simulink library "se2a_command_lib"  (R2018b)
settings: Solver=VariableStepAuto  StartTime=0.0  StopTime=10.0  RelTol=1e-3
undefined symbols (not defined in the file): aircraft
libraries: unit_conversions_lib x5, $bdroot x1
settings Model: Creator=Ybeyer  LastModifiedBy=cava_da
settings SFSimCC: SimUseLocalCustomCode=off
settings RTWCC: RTWUseLocalCustomCode=off
settings CodeAppCC: StateflowObjectComments=on

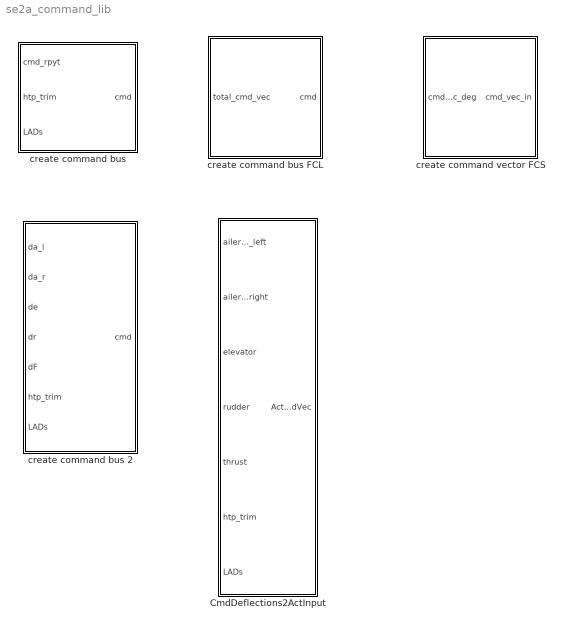
== system se2a_command_lib ==
  CmdDeflections2ActInput : Subsystem  mask{actuators=aircraft.actuators}
      mask prompts: actuators "Actuator parameters"
  create command bus : Subsystem  mask{num_ailerons=aircraft.wing_main.params.num_flaps/2}
      mask prompts: num_ailerons "Number of ailerons per side"
      mask DialogControl DescGroupVar Prompt: Create command bus
  create command bus 2 : Subsystem
      mask DialogControl DescGroupVar Prompt: Create command bus
  create command bus FCL : Subsystem  mask{n_ail_pairs=aircraft.wing_main.params.num_flaps/2, n_LADs=aircraft.wing_main.params.num_lads}
      mask prompts: n_ail_pairs "Number of aileron pairs"; n_LADs "Number of LADs"
      mask DialogControl DescGroupVar Prompt: Create command bus
  create command vector FCS : Subsystem  mask{n_ail_pairs=aircraft.wing_main.params.num_flaps/2, n_LADs=aircraft.wing_main.params.num_lads}
      mask prompts: n_ail_pairs "Number of aileron pairs"; n_LADs "Number of LADs"
      mask DialogControl DescGroupVar Prompt: Create command bus

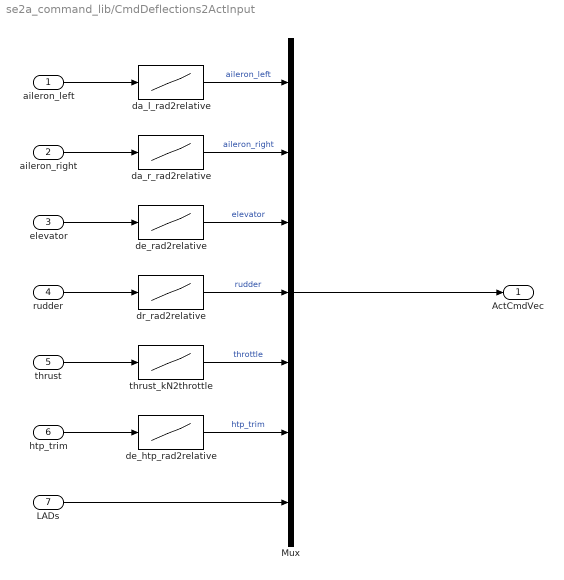
== system se2a_command_lib/CmdDeflections2ActInput ==
  aileron_left : Inport
  aileron_right : Inport  Port=2
  elevator : Inport  Port=3
  rudder : Inport  Port=4
  thrust : Inport  Port=5
  htp_trim : Inport  Port=6
  LADs : Inport  Port=7
  Mux : Mux  Inputs=7
  da_l_rad2relative : Lookup_n-D  NumberOfTableDimensions=1  BreakpointsForDimension1=[actuators.aileron.defl_min,actuators.aileron.defl_max]  Table=[-1,1]  ExtrapMethod=Clip  InternalRulePriority=Speed  RndMeth=Simplest  InputSameDT=on
  da_r_rad2relative : Lookup_n-D  NumberOfTableDimensions=1  BreakpointsForDimension1=[actuators.aileron.defl_min,actuators.aileron.defl_max]  Table=[-1,1]  ExtrapMethod=Clip  InternalRulePriority=Speed  RndMeth=Simplest  InputSameDT=on
  de_htp_rad2relative : Lookup_n-D  NumberOfTableDimensions=1  BreakpointsForDimension1=[actuators.htp_trim.defl_min,actuators.htp_trim.defl_max]  Table=[-1,1]  ExtrapMethod=Clip  InternalRulePriority=Speed  RndMeth=Simplest  InputSameDT=on
  de_rad2relative : Lookup_n-D  NumberOfTableDimensions=1  BreakpointsForDimension1=[actuators.elevator.defl_min,actuators.elevator.defl_max]  Table=[-1,1]  ExtrapMethod=Clip  InternalRulePriority=Speed  RndMeth=Simplest  InputSameDT=on
  dr_rad2relative : Lookup_n-D  NumberOfTableDimensions=1  BreakpointsForDimension1=[actuators.rudder.defl_min,actuators.rudder.defl_max]  Table=[-1,1]  ExtrapMethod=Clip  InternalRulePriority=Speed  RndMeth=Simplest  InputSameDT=on
  thrust_kN2throttle : Lookup_n-D  NumberOfTableDimensions=1  BreakpointsForDimension1=[0,actuators.engines.thrust_max]  Table=[0,1]  ExtrapMethod=Clip  InternalRulePriority=Speed  RndMeth=Simplest  InputSameDT=on
  ActCmdVec : Outport
  wires:
  LADs/1 -> Mux/7
  rudder/1 -> dr_rad2relative/1
  htp_trim/1 -> de_htp_rad2relative/1
  aileron_right/1 -> da_r_rad2relative/1
  Mux/1 -> ActCmdVec/1
  thrust/1 -> thrust_kN2throttle/1
  elevator/1 -> de_rad2relative/1
  de_rad2relative/1 -> Mux/3  "elevator"
  de_htp_rad2relative/1 -> Mux/6  "htp_trim"
  dr_rad2relative/1 -> Mux/4  "rudder"
  da_l_rad2relative/1 -> Mux/1  "aileron_left"
  thrust_kN2throttle/1 -> Mux/5  "throttle"
  da_r_rad2relative/1 -> Mux/2  "aileron_right"
  aileron_left/1 -> da_l_rad2relative/1

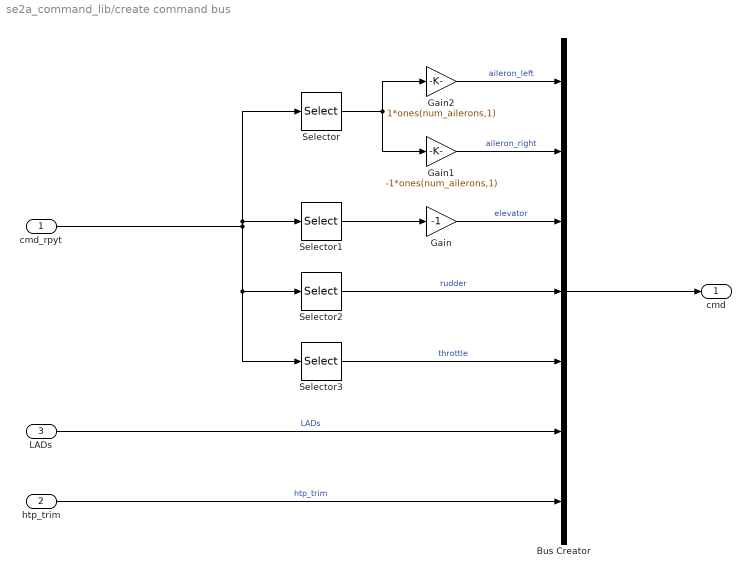
== system se2a_command_lib/create command bus ==
  cmd_rpyt : Inport
  htp_trim : Inport  Port=2
  LADs : Inport  Port=3
  Bus Creator : BusCreator  Inputs=7
  Gain : Gain  Gain=-1
  Gain1 : Gain  Gain=-1*ones(num_ailerons,1)
  Gain2 : Gain  Gain=1*ones(num_ailerons,1)
  Selector : Selector  InputPortWidth=4  IndexOptions=Index vector (dialog)  Indices=1  OutputSizes=1
  Selector1 : Selector  InputPortWidth=4  IndexOptions=Index vector (dialog)  Indices=2  OutputSizes=1
  Selector2 : Selector  InputPortWidth=4  IndexOptions=Index vector (dialog)  Indices=3  OutputSizes=1
  Selector3 : Selector  InputPortWidth=4  IndexOptions=Index vector (dialog)  Indices=4  OutputSizes=1
  cmd : Outport
  wires:
  cmd_rpyt/1 -> Selector/1, Selector1/1, Selector3/1, Selector2/1
  Bus Creator/1 -> cmd/1
  LADs/1 -> Bus Creator/6  "LADs"
  Selector/1 -> Gain1/1, Gain2/1
  Selector1/1 -> Gain/1
  Selector2/1 -> Bus Creator/4  "rudder"
  Selector3/1 -> Bus Creator/5  "throttle"
  Gain/1 -> Bus Creator/3  "elevator"
  Gain1/1 -> Bus Creator/2  "aileron_right"
  htp_trim/1 -> Bus Creator/7  "htp_trim"
  Gain2/1 -> Bus Creator/1  "aileron_left"

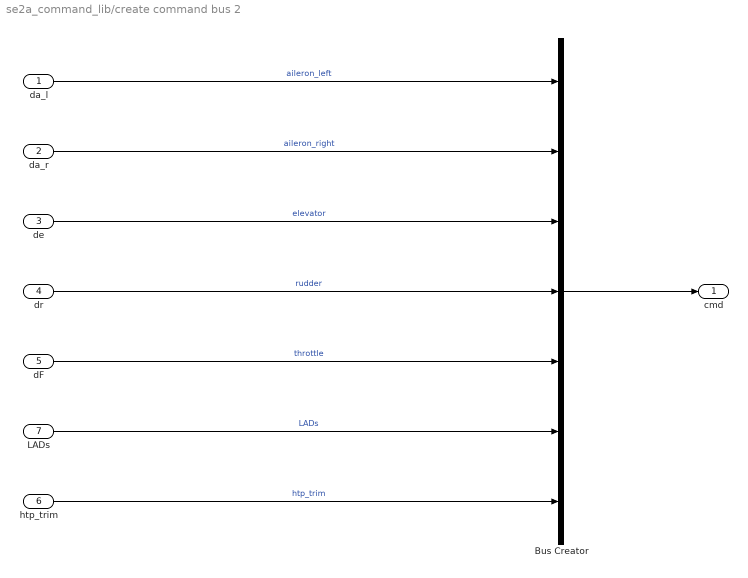
== system se2a_command_lib/create command bus 2 ==
  da_l : Inport
  da_r : Inport  Port=2
  de : Inport  Port=3
  dr : Inport  Port=4
  dF : Inport  Port=5
  htp_trim : Inport  Port=6
  LADs : Inport  Port=7
  Bus Creator : BusCreator  Inputs=7
  cmd : Outport
  wires:
  htp_trim/1 -> Bus Creator/7  "htp_trim"
  da_r/1 -> Bus Creator/2  "aileron_right"
  de/1 -> Bus Creator/3  "elevator"
  dF/1 -> Bus Creator/5  "throttle"
  dr/1 -> Bus Creator/4  "rudder"
  da_l/1 -> Bus Creator/1  "aileron_left"
  LADs/1 -> Bus Creator/6  "LADs"
  Bus Creator/1 -> cmd/1

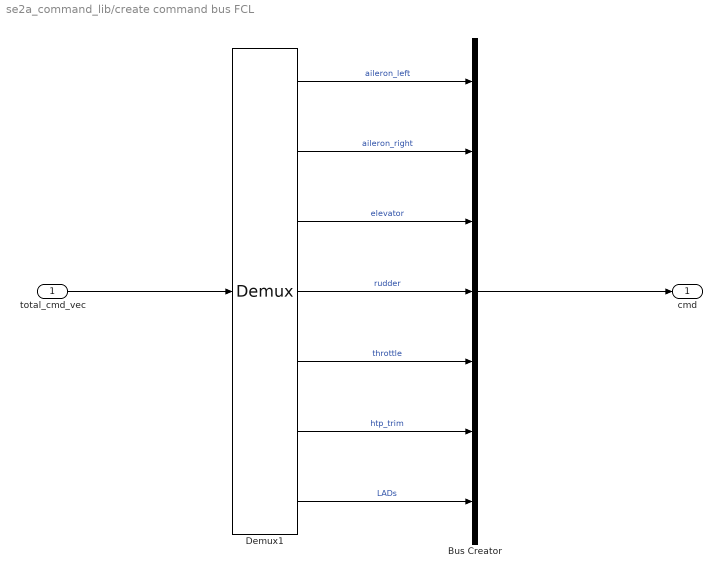
== system se2a_command_lib/create command bus FCL ==
  total_cmd_vec : Inport
  Bus Creator : BusCreator  Inputs=7
  Demux1 : Demux  Outputs=[n_ail_pairs, n_ail_pairs, 1, 1, 1, 1, n_LADs]
  cmd : Outport
  wires:
  total_cmd_vec/1 -> Demux1/1
  Demux1/7 -> Bus Creator/7  "LADs"
  Demux1/6 -> Bus Creator/6  "htp_trim"
  Demux1/4 -> Bus Creator/4  "rudder"
  Demux1/5 -> Bus Creator/5  "throttle"
  Demux1/3 -> Bus Creator/3  "elevator"
  Demux1/2 -> Bus Creator/2  "aileron_right"
  Demux1/1 -> Bus Creator/1  "aileron_left"
  Bus Creator/1 -> cmd/1

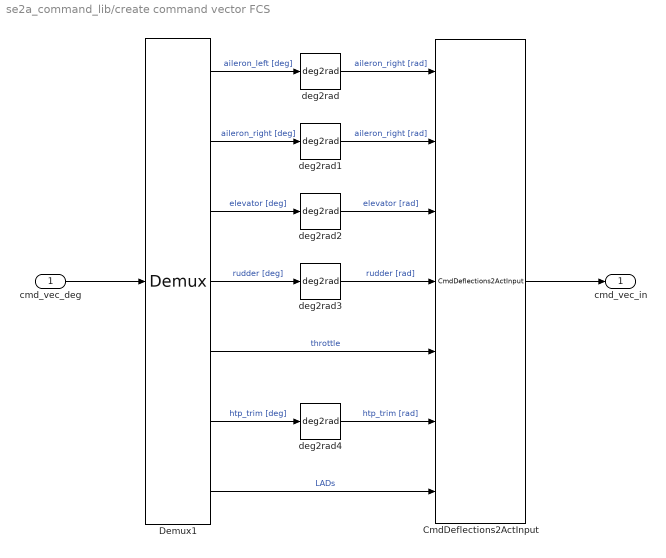
== system se2a_command_lib/create command vector FCS ==
  cmd_vec_deg : Inport
  CmdDeflections2ActInput : $bdroot/CmdDeflections2ActInput  actuators=aircraft.actuators
  Demux1 : Demux  Outputs=[n_ail_pairs, n_ail_pairs, 1, 1, 1, 1, n_LADs]
  deg2rad{,1..4} (5 alike) : unit_conversions_lib/deg2rad
      settings: SourceProductName=LADAC
  cmd_vec_in : Outport
  wires:
  CmdDeflections2ActInput/1 -> cmd_vec_in/1
  Demux1/1 -> deg2rad/1  "aileron_left [deg]"
  Demux1/2 -> deg2rad1/1  "aileron_right [deg]"
  Demux1/3 -> deg2rad2/1  "elevator [deg]"
  Demux1/5 -> CmdDeflections2ActInput/5  "throttle"
  Demux1/4 -> deg2rad3/1  "rudder [deg]"
  Demux1/6 -> deg2rad4/1  "htp_trim [deg]"
  Demux1/7 -> CmdDeflections2ActInput/7  "LADs"
  cmd_vec_deg/1 -> Demux1/1
  deg2rad/1 -> CmdDeflections2ActInput/1  "aileron_right [rad]"
  deg2rad1/1 -> CmdDeflections2ActInput/2  "aileron_right [rad]"
  deg2rad2/1 -> CmdDeflections2ActInput/3  "elevator [rad]"
  deg2rad3/1 -> CmdDeflections2ActInput/4  "rudder [rad]"
  deg2rad4/1 -> CmdDeflections2ActInput/6  "htp_trim [rad]"
